simulink model "stackercrane_singlemass_verification_validation"  (R2020b)
settings: Solver=ode45  StartTime=0.0  StopTime=15  MaxStep=0.02  RelTol=1e-3  EnableMultiTasking=on
settings Model: Creator=beck  LastModifiedBy=Iris
settings DataIOCC: LimitDataPoints=on  SaveFormat=Array  SignalLoggingSaveFormat=ModelDataLogs  ReturnWorkspaceOutputs=off
settings OptimizationCC: ExpressionDepthLimit=2147483647  InitFltsAndDblsToZero=on  LifeSpan=inf
settings DebuggingCC: SaveWithParameterizedLinksMsg=none  UnderspecifiedInitializationDetection=Classic  MergeDetectMultiDrivingBlocksExec=none  SignalResolutionControl=TryResolveAllWithWarning  SolverPrmCheckMsg=warning  FcnCallInpInsideContextMsg=warning  StateNameClashWarn=warning  SFUnexpectedBacktrackingDiag=warning  SFNoUnconditionalDefaultTransitionDiag=warning  SFExecutionAtInitializationDiag=none  ArithmeticOperatorsInVariantConditions=warning
settings HardwareCC: ProdBitPerPointer=32  ProdBitPerSizeT=32  ProdBitPerPtrDiffT=32  ProdLargestAtomicFloat=None  ProdIntDivRoundTo=Undefined  ProdEndianess=Unspecified  ProdWordSize=32  ProdHWDeviceType=32-bit Generic
settings ModelReferenceCC: PropagateSignalLabelsOutOfModel=off
settings SFSimCC: SimUseLocalCustomCode=off  CustomCodeUndefinedFunction=UseInterfaceOnly
settings RTWCC: RTWUseLocalCustomCode=off
settings CodeAppCC: StateflowObjectComments=on
settings GRTTargetCC: TargetFcnLib=ansi_tfl_tmw.mat  TargetLangStandard=C89/C90 (ANSI)  CombineOutputUpdateFcns=off  GRTInterface=on
settings ConfigComp: CovMetricSettings=dw  CovSaveCumulativeToWorkspaceVar=on  CovSaveSingleToWorkspaceVar=on  CovExternalEMLEnable=off

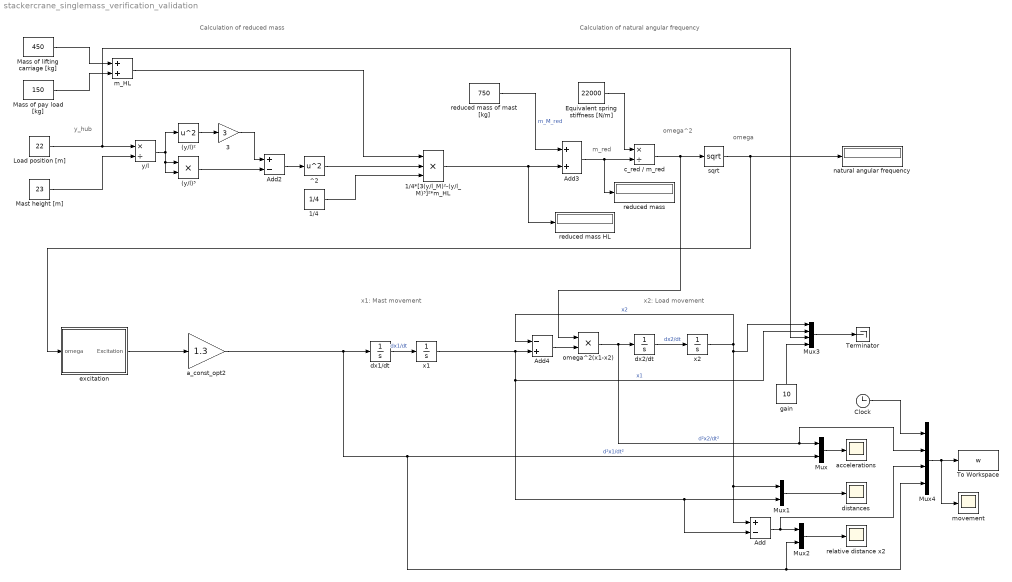
== system stackercrane_singlemass_verification_validation ==
  note: y_hub
  note: m_red
  note: omega^2
  note: omega
  note: Calculation of reduced mass
  note: Calculation of natural angular frequency
  note: x1: Mast movement
  note: x2: Load movement
  (y/l)² : Math  Operator=square  SignedPower=on  SaturateOnIntegerOverflow=on
  (y/l)³ : Product  RndMeth=Zero
  1/4 : Constant  Value=1/4
  1/4*[3(y/l_M)²-(y/l_M)³]²*m_HL : Product  Inputs=3  RndMeth=Zero
  3 : Gain  Gain=3
  Add : Sum  Inputs=+-
  Add2 : Sum  Inputs=+-
  Add3 : Sum
  Add4 : Sum  Inputs=-+
  Clock : Clock
  Equivalent spring stiffness [N/m] : Constant  Value=22000
  Load position [m] : Constant  Value=22
  Mass of lifting carriage [kg] : Constant  Value=450
  Mass of pay load [kg] : Constant  Value=150
  Mast height [m] : Constant  Value=23
  Mux : Mux  Inputs=2
  Mux1 : Mux  Inputs=2
  Mux2 : Mux  Inputs=2
  Mux3 : Mux
  Mux4 : Mux
  Terminator : Terminator
  To Workspace : ToWorkspace  VariableName=w  SampleTime=-1
  ^2 : Math  Operator=square  SignedPower=on  SaturateOnIntegerOverflow=on
  a_const_opt2 : Gain  Gain=1.3
  accelerations : Scope
  c_red / m_red : Product  Inputs=*/  RndMeth=Zero
  distances : Scope
  dx1/dt : Integrator
  dx2/dt : Integrator
  excitation : Subsystem
  gain : Constant  Value=10
  m_HL : Sum
  movement : Scope
  natural angular frequency : Display
  omega^2(x1-x2) : Product  RndMeth=Zero
  reduced mass : Display
      settings: Decimation=2
  reduced mass HL : Display
      settings: Decimation=2
  reduced mass of mast [kg] : Constant  Value=750
  relative distance x2 : Scope
  sqrt : Math  Operator=sqrt  SignedPower=on  SaturateOnIntegerOverflow=on
  x1 : Integrator
  x2 : Integrator
  y/l : Product  Inputs=*/  RndMeth=Zero
  wires:
  Load position [m]/1 -> y/l/1, Mux3/3
  Mux/1 -> accelerations/1
  Mux1/1 -> distances/1
  Mast height [m]/1 -> y/l/2
  (y/l)²/1 -> 3/1
  3/1 -> Add2/1
  (y/l)³/1 -> Add2/2
  y/l/1 -> (y/l)³/2, (y/l)³/1, (y/l)²/1
  Equivalent spring stiffness [N/m]/1 -> c_red / m_red/1
  c_red / m_red/1 -> sqrt/1, omega^2(x1-x2)/1
  Add3/1 -> reduced mass/1, c_red / m_red/2
  sqrt/1 -> natural angular frequency/1, excitation/1(omega)
  omega^2(x1-x2)/1 -> dx2/dt/1, Mux/1, Mux4/2  "d²x2/dt²"
  dx2/dt/1 -> x2/1  "dx2/dt"
  dx1/dt/1 -> x1/1  "dx1/dt"
  Add4/1 -> omega^2(x1-x2)/2
  x1/1 -> Add4/2, Mux1/2, Add/2, Mux3/2  "x1"
  x2/1 -> Add4/1, Add/1, Mux1/1, Mux3/1  "x2"
  gain/1 -> Mux3/4
  Add2/1 -> ^2/1
  reduced mass of mast [kg]/1 -> Add3/1  "m_M_red"
  Mux2/1 -> relative distance x2/1
  Add/1 -> Mux2/1, Mux4/3
  Mass of pay load [kg]/1 -> m_HL/2
  Mass of lifting carriage [kg]/1 -> m_HL/1
  1/4*[3(y/l_M)²-(y/l_M)³]²*m_HL/1 -> Add3/2, reduced mass HL/1
  ^2/1 -> 1/4*[3(y/l_M)²-(y/l_M)³]²*m_HL/2
  m_HL/1 -> 1/4*[3(y/l_M)²-(y/l_M)³]²*m_HL/1
  1/4/1 -> 1/4*[3(y/l_M)²-(y/l_M)³]²*m_HL/3
  a_const_opt2/1 -> dx1/dt/1, Mux/2, Mux2/2, Mux4/4  "d²x1/dt²"
  excitation/1(Excitation) -> a_const_opt2/1
  Clock/1 -> Mux4/1
  Mux4/1 -> To Workspace/1, movement/1
  Mux3/1 -> Terminator/1

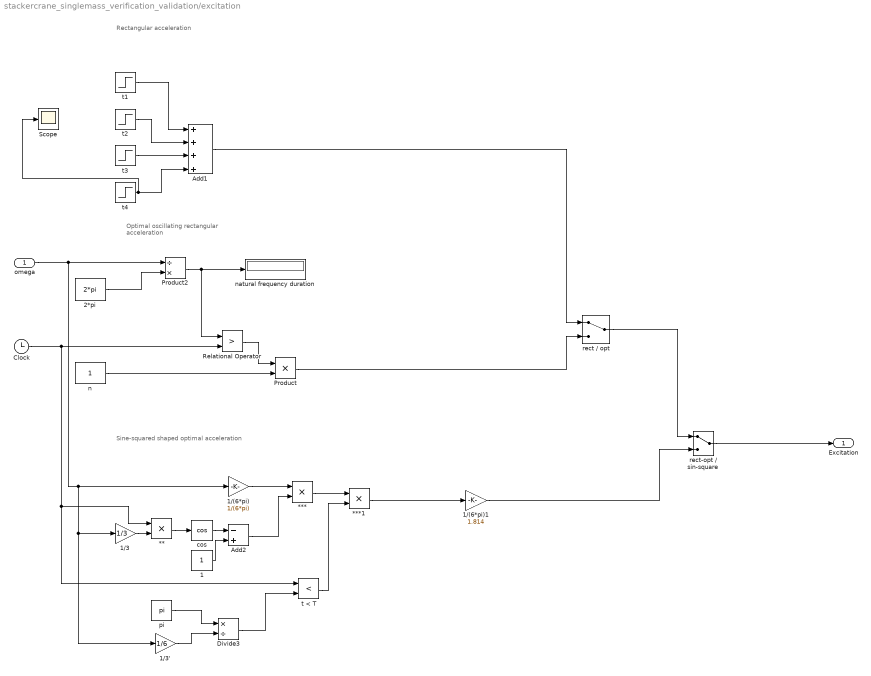
== system stackercrane_singlemass_verification_validation/excitation ==
  note: Sine-squared shaped optimal acceleration
  note: Optimal oscillating rectangular acceleration
  note: Rectangular acceleration
  omega : Inport
  ** : Product  RndMeth=Zero
  *** : Product  RndMeth=Zero
  ***1 : Product  RndMeth=Zero
  1 : Constant
  1/(6*pi) : Gain  Gain=1/(6*pi)
  1/(6*pi)1 : Gain  Gain=1.814
  1/3 : Gain  Gain=1/3
  1/3' : Gain  Gain=1/6
  2*pi : Constant  Value=2*pi
  Add1 : Sum  Inputs=++++
  Add2 : Sum  Inputs=-+
  Clock : Clock
  Divide3 : Product  Inputs=*/
  Product : Product  RndMeth=Zero
  Product2 : Product  Inputs=/*  RndMeth=Zero
  Relational Operator : RelationalOperator  Operator=>  RndMeth=Nearest
  Scope : Scope
  "cos " : Trigonometry  Operator=cos
  n : Constant
  natural frequency duration : Display
  pi : Constant  Value=pi
  rect / opt : ManualSwitch
  rect-opt / sin-square : ManualSwitch
  t < T : RelationalOperator  Operator=<  OutDataTypeStr=boolean  RndMeth=Nearest
  t1 : Step  Time=2  SampleTime=0
  t2 : Step  Time=4  After=-1  SampleTime=0
  t3 : Step  Time=10  After=-1  SampleTime=0
  t4 : Step  Time=12  SampleTime=0
  Excitation : Outport
  wires:
  2*pi/1 -> Product2/2
  t1/1 -> Add1/1
  t2/1 -> Add1/2
  Clock/1 -> Relational Operator/2, **/1, t < T/1
  n/1 -> Product/2
  t3/1 -> Add1/3
  t4/1 -> Scope/1, Add1/4
  Product2/1 -> natural frequency duration/1, Relational Operator/1
  Relational Operator/1 -> Product/1
  Product/1 -> rect / opt/2
  omega/1 -> Product2/1, 1/(6*pi)/1, 1/3/1, 1/3'/1
  1/3/1 -> **/2
  **/1 -> "cos "/1
  "cos "/1 -> Add2/1
  1/1 -> Add2/2
  1/(6*pi)/1 -> ***/1
  Add2/1 -> ***/2
  ***/1 -> ***1/1
  pi/1 -> Divide3/1
  Divide3/1 -> t < T/2
  t < T/1 -> ***1/2
  rect-opt / sin-square/1 -> Excitation/1
  1/3'/1 -> Divide3/2
  ***1/1 -> 1/(6*pi)1/1
  1/(6*pi)1/1 -> rect-opt / sin-square/2
  Add1/1 -> rect / opt/1
  rect / opt/1 -> rect-opt / sin-square/1
